simulink model "POINTING"  (R2025b)
settings: Solver=ode45  StartTime=0.0  StopTime=20  RelTol=1e-3
values from neighbouring files (symbols this model uses):
  J = 0.002    [SIMULINK_InitialParameters.m]
  Jw = 1e-5    (= 1e-05)    [SIMULINK_InitialParameters.m]
  Kd = 0.01    [SIMULINK_InitialParameters.m]
  Kp = 0.02    [SIMULINK_InitialParameters.m]
  omega0 = deg2rad(8)    [SIMULINK_InitialParameters.m]
  omega_w0 = 0    [SIMULINK_InitialParameters.m]
  theta0 = deg2rad(15)    [SIMULINK_InitialParameters.m]
  theta_ref = 0    [SIMULINK_InitialParameters.m]
settings Model: Creator=bbtp  LastModifiedBy=bbtp

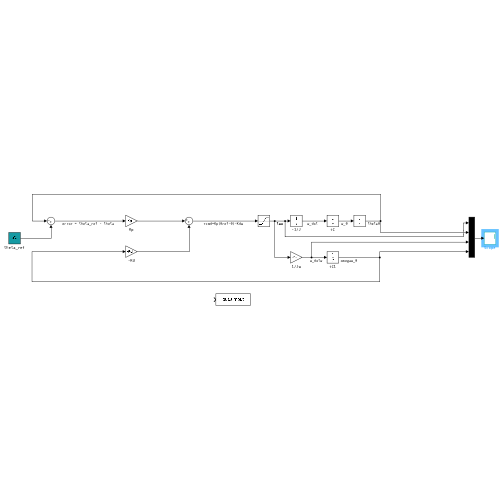
[thumbnail: Simulink's stored preview of the top-level diagram]
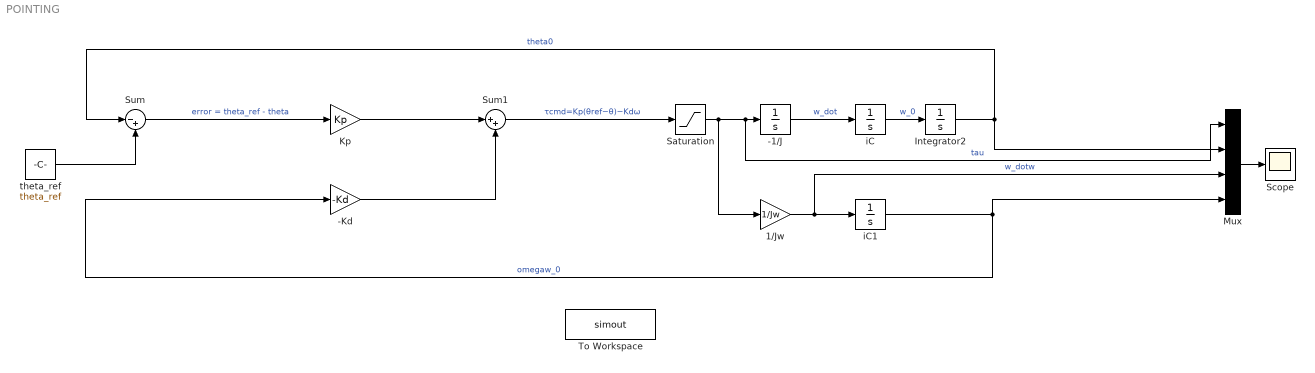
== system POINTING ==
  -1/J : Integrator  InitialCondition=-1/J
  -Kd : Gain  Gain=-Kd
  1/Jw : Gain  Gain=1/Jw
  Integrator2 : Integrator  InitialCondition=theta0
  Kp : Gain  Gain=Kp
  Mux : Mux
  Saturation : Saturate
  Scope : Scope
      settings: ActiveDisplayYMinimum=-137401.46386583507  ActiveDisplayYMaximum=237310.02608480997
  Sum : Sum  Inputs=|-+
  Sum1 : Sum  Inputs=|++
  To Workspace : ToWorkspace  VariableName=simout  SaveFormat=Timeseries  SampleTime=-1
  iC : Integrator  InitialCondition=omega0
  iC1 : Integrator  InitialCondition=omega_w0
  theta_ref : Constant  Value=theta_ref
  wires:
  Sum/1 -> Kp/1  "error = theta_ref - theta"
  Kp/1 -> Sum1/1
  -Kd/1 -> Sum1/2
  Sum1/1 -> Saturation/1  "τcmd​=Kp​(θref​−θ)−Kd​ω"
  Saturation/1 -> 1/Jw/1, Mux/1, -1/J/1  "tau"
  -1/J/1 -> iC/1  "w_dot"
  iC/1 -> Integrator2/1  "w_0"
  theta_ref/1 -> Sum/2
  Integrator2/1 -> Sum/1, Mux/2  "theta0"
  1/Jw/1 -> Mux/3, iC1/1  "w_dotw"
  iC1/1 -> -Kd/1, Mux/4  "omegaw_0"
  Mux/1 -> Scope/1
